simulink model "projekt1_9"  (R2016b)
settings: Solver=VariableStepAuto  StartTime=0.0  StopTime=100  RelTol=1e-3
values from neighbouring files (symbols this model uses):
  Tp = 1    [projekt1.m]    (also in projekt1_5.m)
  u_ = 2    [projekt1.m]    (also in projekt1_5.m = 0)
settings Model: Creator=m  LastModifiedBy=m

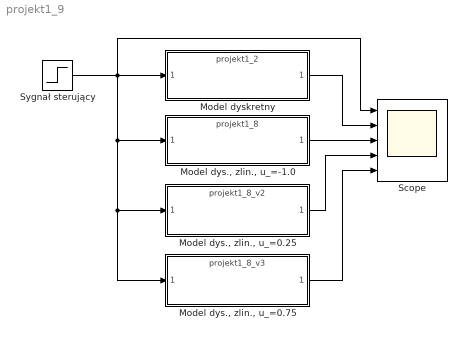
== system projekt1_9 ==
  "Model dys., zlin., u_=-1.0" : ModelReference  ModelNameDialog=projekt1_8  SimulationMode=Normal  ModelReferenceVersion=1.12
  "Model dys., zlin., u_=0.25" : ModelReference  ModelNameDialog=projekt1_8_v2  SimulationMode=Normal  ModelReferenceVersion=1.15
  "Model dys., zlin., u_=0.75" : ModelReference  ModelNameDialog=projekt1_8_v3  SimulationMode=Normal  ModelReferenceVersion=1.15
  Model dyskretny : ModelReference  ModelNameDialog=projekt1_2  SimulationMode=Normal  ModelReferenceVersion=1.6
  Scope : Scope  NumInputPorts=5
  Sygnał sterujący : Step  After=u_  SampleTime=Tp
  wires:
  Sygnał sterujący/1 -> Scope/1, Model dyskretny/1, "Model dys., zlin., u_=-1.0"/1, "Model dys., zlin., u_=0.25"/1, "Model dys., zlin., u_=0.75"/1
  "Model dys., zlin., u_=-1.0"/1 -> Scope/3
  "Model dys., zlin., u_=0.75"/1 -> Scope/5
  "Model dys., zlin., u_=0.25"/1 -> Scope/4
  Model dyskretny/1 -> Scope/2
